simulink subsystem "ActiveSuspensionControl"  (R2025b)
settings: Solver=VariableStepAuto  StartTime=0.0  StopTime=10.0  RelTol=1e-3
settings Model: Creator=Murl0  LastModifiedBy=Murl0

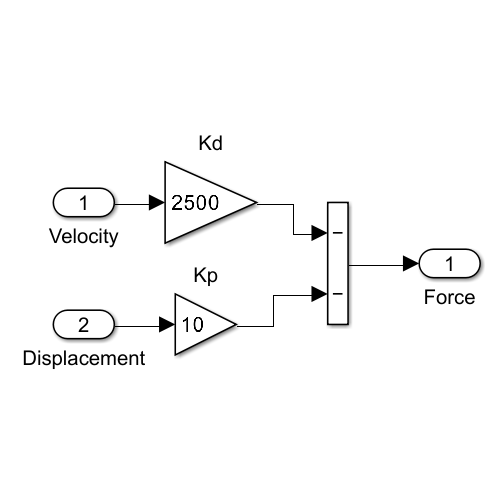
[thumbnail: Simulink's stored preview of the top-level diagram]
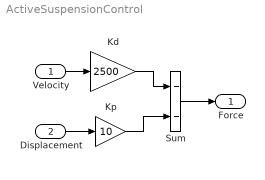
== system ActiveSuspensionControl ==
  Velocity : Inport
  Displacement : Inport  Port=2
  Kd : Gain  Gain=2500
  Kp : Gain  Gain=10
  Sum : Sum  Inputs=--
  Force : Outport
  wires:
  Velocity/1 -> Kd/1
  Displacement/1 -> Kp/1
  Kd/1 -> Sum/1
  Kp/1 -> Sum/2
  Sum/1 -> Force/1
